simulink model "InductionCookerStateFlow"  (R2023a)
settings: Solver=FixedStepDiscrete  StartTime=0.0  StopTime=2000  FixedStep=0.1  RelTol=1e-3  EnableMultiTasking=on
settings Model: Creator=antonio  LastModifiedBy=antonio
settings SolverCC: AlgebraicLoopSolver=TrustRegion  AutoInsertRateTranBlk=on
settings DataIOCC: LimitDataPoints=on
settings OptimizationCC: LifeSpan=inf
settings DebuggingCC: UnconnectedInputMsg=warning  UnconnectedOutputMsg=warning  UnconnectedLineMsg=warning  AllowSymbolicDim=off  SFUnexpectedBacktrackingDiag=warning  SFNoUnconditionalDefaultTransitionDiag=warning  SFExecutionAtInitializationDiag=none  ArithmeticOperatorsInVariantConditions=warning
settings ModelReferenceCC: EnableRefExpFcnMdlSchedulingChecks=on
settings SFSimCC: SimUseLocalCustomCode=off  CustomCodeUndefinedFunction=UseInterfaceOnly
settings RTWCC: RTWUseLocalCustomCode=off  DLArmComputeVersion=19.05
settings CodeAppCC: StateflowObjectComments=on
settings GRTTargetCC: TargetLangStandard=C89/C90 (ANSI)
settings ConfigComp: CovMetricSettings=dw  CovSaveCumulativeToWorkspaceVar=on  CovSaveSingleToWorkspaceVar=on  CovExternalEMLEnable=off  CovSFcnEnable=off

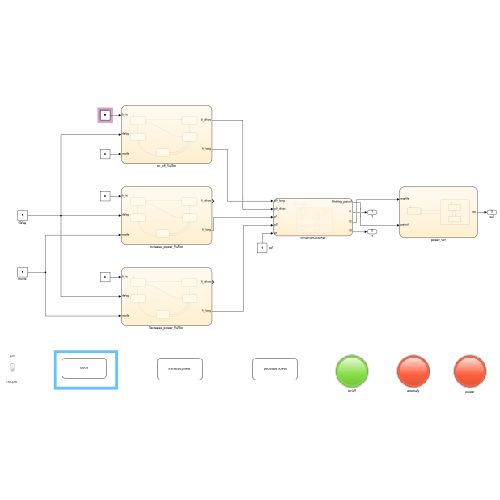
[thumbnail: Simulink's stored preview of the top-level diagram]
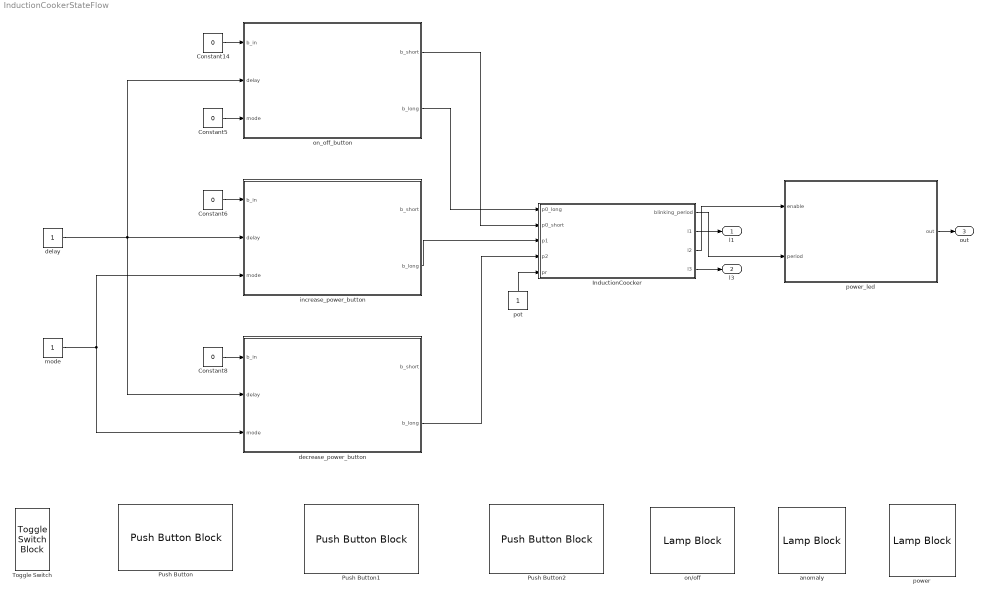
== system InductionCookerStateFlow ==
  Constant{5..6,8,14} (4 alike) : Constant  Value=0  OutDataTypeStr=boolean
  InductionCoocker : Stateflow chart  TreatAsAtomicUnit=on
  Push Button : PushButtonBlock  ButtonText=on/off  OffValue=0.000000
  Push Button1 : PushButtonBlock  ButtonText=increase power  OffValue=0.000000
  Push Button2 : PushButtonBlock  ButtonText=decrease power  OffValue=0.000000
  Toggle Switch : ToggleSwitchBlock  LabelPosition=Hide
      settings: Values={{'not pot', 'pot'}, [0 1]}
  anomaly : LampBlock  LabelPosition=Hide
  "decrease_power_button " : Stateflow chart  TreatAsAtomicUnit=on
  delay : Constant
  increase_power_button : Stateflow chart  TreatAsAtomicUnit=on
  mode : Constant  OutDataTypeStr=boolean
  on/off : LampBlock  LabelPosition=Hide
  on_off_button : Stateflow chart  TreatAsAtomicUnit=on
  pot : Constant  OutDataTypeStr=boolean
  power : LampBlock  LabelPosition=Hide
  power_led : Stateflow chart  TreatAsAtomicUnit=on
  l1 : Outport
  l3 : Outport  Port=2
  out : Outport  Port=3
  wires:
  on_off_button/1(b_short) -> InductionCoocker/2(p0_short)
  on_off_button/2(b_long) -> InductionCoocker/1(p0_long)
  increase_power_button/2(b_long) -> InductionCoocker/3(p1)
  "decrease_power_button "/2(b_long) -> InductionCoocker/4(p2)
  InductionCoocker/1(blinking_period) -> power_led/2(period)
  InductionCoocker/3(l2) -> power_led/1(enable)
  power_led/1(out) -> out/1
  InductionCoocker/2(l1) -> l1/1
  InductionCoocker/4(l3) -> l3/1
  Constant5/1 -> on_off_button/3(mode)
  mode/1 -> increase_power_button/3(mode), "decrease_power_button "/3(mode)
  delay/1 -> "decrease_power_button "/2(delay), increase_power_button/2(delay), on_off_button/2(delay)
  Constant14/1 -> on_off_button/1(b_in)
  Constant6/1 -> increase_power_button/1(b_in)
  Constant8/1 -> "decrease_power_button "/1(b_in)
  pot/1 -> InductionCoocker/5(pr)

== stateflow chart InductionCookerStateFlow/on_off_button ==
  state wait_pressed
    en: b_short = RELEASED;
    b_long = RELEASED
  state pressed
    en: b_short = PRESSED
  state wait_longpressed
    en: b_short = RELEASED
  state wait_released
    en: b_long = RELEASED
  state longpressed
    on after(delay, sec):
    b_long = PRESSED;
  (default) -> wait_pressed
  wait_pressed -> pressed [order 1] : [mode == 0 & b_in == PRESSED]
  wait_pressed -> wait_longpressed [order 2] : [mode == 1]
  pressed -> wait_longpressed : [b_in == RELEASED]
  wait_released -> wait_pressed : [b_in == RELEASED]
  longpressed -> wait_released [order 1] : [b_long == PRESSED & b_in == PRESSED]
  wait_longpressed -> longpressed : [b_in == PRESSED]
  longpressed -> wait_longpressed [order 2] : [b_in == RELEASED]
  data: b_in input boolean; delay input; b_short output boolean; b_long output boolean; PRESSED constant boolean =true; RELEASED constant boolean =false; mode input boolean

== stateflow chart InductionCookerStateFlow/decrease_power_button  ==
  state wait_pressed
    en: b_short = RELEASED;
    b_long = RELEASED
  state pressed
    en: b_short = PRESSED
  state wait_longpressed
    en: b_short = RELEASED
  state wait_released
    en: b_long = RELEASED
  state longpressed
    on after(delay, sec):
    b_long = PRESSED;
  (default) -> wait_pressed
  wait_pressed -> pressed [order 1] : [mode == 0 & b_in == PRESSED]
  wait_pressed -> wait_longpressed [order 2] : [mode == 1]
  pressed -> wait_longpressed : [b_in == RELEASED]
  wait_released -> wait_pressed : [b_in == RELEASED]
  longpressed -> wait_released [order 1] : [b_long == PRESSED & b_in == PRESSED]
  wait_longpressed -> longpressed : [b_in == PRESSED]
  longpressed -> wait_longpressed [order 2] : [b_in == RELEASED]
  data: b_in input boolean; delay input; b_short output boolean; b_long output boolean; PRESSED constant boolean =true; RELEASED constant boolean =false; mode input boolean

== stateflow chart InductionCookerStateFlow/increase_power_button ==
  state wait_pressed
    en: b_short = RELEASED;
    b_long = RELEASED
  state pressed
    en: b_short = PRESSED
  state wait_longpressed
    en: b_short = RELEASED
  state wait_released
    en: b_long = RELEASED
  state longpressed
    on after(delay, sec):
    b_long = PRESSED;
  (default) -> wait_pressed
  wait_pressed -> pressed [order 1] : [mode == 0 & b_in == PRESSED]
  wait_pressed -> wait_longpressed [order 2] : [mode == 1]
  pressed -> wait_longpressed : [b_in == RELEASED]
  wait_released -> wait_pressed : [b_in == RELEASED]
  longpressed -> wait_released [order 1] : [b_long == PRESSED & b_in == PRESSED]
  wait_longpressed -> longpressed : [b_in == PRESSED]
  longpressed -> wait_longpressed [order 2] : [b_in == RELEASED]
  data: b_in input boolean; delay input; b_short output boolean; b_long output boolean; PRESSED constant boolean =true; RELEASED constant boolean =false; mode input boolean

== stateflow chart InductionCookerStateFlow/power_led ==
  state blink
    state blink_on
      en: out = ACTIVE
    state blink_off
      en: out = DISACTIVE
    (default) -> blink_on
    blink_off -> blink_on : after(period, msec)
    blink_on -> blink_off : after(period, msec)
  state off
    en: out = DISACTIVE;
  (default) -> off
  off -> blink : [enable == ACTIVE]
  blink -> off : [enable == DISACTIVE]
  data: enable input boolean; out output boolean; ACTIVE constant boolean =true; DISACTIVE constant boolean =false; period input

== stateflow chart InductionCookerStateFlow/InductionCoocker ==
  state off
    en: l1 = OFF; l2 = OFF, l3 = OFF
  state inactive
    en: l1 = ON; l2 = OFF; err_status = ~ERR
  state active
    state powers [parallel]
      settings: executionOrder=1
      state waiting_inactive
      state power_500w
        state waiting_500w
        state working_500w
          en: l2 = ON;
          blinking_period = DELAY_500;
        (default) -> waiting_500w
        waiting_500w -> working_500w : after(POWER_DELAY, sec)[pr == POT_IS_PRESENT]
      state power_300w
        state waiting_300w
        state working_300w
          en: l2 = ON;
          blinking_period = DELAY_300;
        (default) -> waiting_300w
        waiting_300w -> working_300w : after(POWER_DELAY, sec)[pr == POT_IS_PRESENT]
      state power_1500w
        state waiting_1500w
        state working_1500w
          en: l2 = ON;
          blinking_period = DELAY_1500;
        (default) -> waiting_1500w
        waiting_1500w -> working_1500w : after(POWER_DELAY, sec)[pr == POT_IS_PRESENT]
      state power_1000w
        state waiting_1000w
        state working_1000w
          en: l2 = ON;
          blinking_period = DELAY_1000;
        (default) -> waiting_1000w
        waiting_1000w -> working_1000w : after(POWER_DELAY, sec)[pr == POT_IS_PRESENT]
      power_300w -> waiting_inactive [order 1] : [p2 == PRESSED & pr == POT_IS_PRESENT]
      waiting_inactive -> power_300w [order 1] : [p1 == PRESSED & pr == POT_IS_PRESENT]
      (default) -> power_300w
      power_300w -> power_500w [order 2] : [p1 == PRESSED & pr == POT_IS_PRESENT]
      power_500w -> power_300w [order 1] : [p2 == PRESSED & pr == POT_IS_PRESENT]
      power_1000w -> power_500w [order 1] : [p2 == PRESSED & pr == POT_IS_PRESENT]
      power_500w -> power_1000w [order 2] : [p1 == PRESSED & pr == POT_IS_PRESENT]
      power_1500w -> power_1000w : [p2 == PRESSED & pr == POT_IS_PRESENT]
      power_1000w -> power_1500w [order 2] : [p1 == PRESSED & pr == POT_IS_PRESENT]
    state anomaly_guard [parallel]
      settings: executionOrder=2
      state guard
      state anomaly_detected
        en: l3 = ON
        exit: l3 = OFF
      (default) -> guard
      anomaly_detected -> guard [order 2] : after(ANOMALY_DELAY, sec){err_status = ERR}
      anomaly_detected -> guard [order 1] : [pr == POT_IS_PRESENT]
      guard -> anomaly_detected : [pr == ~POT_IS_PRESENT]
  (default) -> off
  off -> inactive : [p0_short == PRESSED]
  active -> inactive [order 1] : [err_status == ERR]
  inactive -> off [order 1] : [p0_long == PRESSED]
  active -> off [order 2] : [p0_long == PRESSED]
  waiting_inactive -> inactive [order 2] : after(POWER_DELAY, sec)
  inactive -> power_300w [order 2] : [p1 == PRESSED & pr == POT_IS_PRESENT]
  data: ERR constant boolean =true; DELAY_300 constant double =2000; p0_long input boolean; p0_short input boolean; p1 input boolean; p2 input boolean; pr input boolean; blinking_period output double; l1 output boolean; l2 output boolean; l3 output boolean; err_status local boolean; ANOMALY_DELAY constant double =10; DELAY_1000 constant double =500; DELAY_1500 constant double =250; DELAY_500 constant double =1000; OFF constant boolean =false; ON constant boolean =true; POT_IS_PRESENT constant boolean =true; PRESSED constant boolean =true; POWER_DELAY constant double =5
